simulink library "line_tracking_algorithm_atomic_sub_chart_library"  (R2013b)
settings: Solver=ode45  StartTime=0.0  StopTime=10.0  RelTol=1e-3
undefined symbols (not defined in the file): DiscIntNeverNeededParam, gcbh, realtime
libraries: legonxtlib x15, simulink x15
(part 2 of 2)

== system line_tracking_algorithm_atomic_sub_chart_library/line_tracking_mode1/line_tracking_mode.LineTrackAltFcn/D ==
  light error : Inport
  Abs1 : Abs
  Constant4 : Constant  Value=[2.5 0]  OutDataTypeStr=single
  Constant5 : Constant  Value=[0 1]  OutDataTypeStr=single
  Discrete Derivative1 : simulink/Discrete/Discrete Derivative  gainval=1.0  ICPrevScaledInput=0.0  InputProcessing=Inherited  OutMin=[]  OutMax=[]  OutDataTypeStr=single  OutputDataTypeScalingMode=single  OutDataType=fixdt(1, 16)  OutScaling=2^-10  DoSatur=off
  Gain2 : Gain  Gain=0.0005
  Low Pass Filter1 : DiscreteFilter  Numerator=[.2]  Denominator=[1 -0.8]
  Product1 : Product  RndMeth=Zero
  Switch1 : Switch
  Volt : Outport
  wires:
  light error/1 -> Low Pass Filter1/1
  Low Pass Filter1/1 -> Discrete Derivative1/1
  Abs1/1 -> Gain2/1
  Constant5/1 -> Switch1/3
  Constant4/1 -> Switch1/1
  Discrete Derivative1/1 -> Switch1/2, Abs1/1
  Switch1/1 -> Product1/1
  Gain2/1 -> Product1/2
  Product1/1 -> Volt/1

== system line_tracking_algorithm_atomic_sub_chart_library/line_tracking_mode1/line_tracking_mode.LineTrackAltFcn/LCD2 ==
  In1 : Inport
  Data Type Conversion : DataTypeConversion  OutDataTypeStr=int32
  LCD : S-Function  FunctionName=nxt_lcd  Parameters=lcdStr1, lcdLine, lcdFormat  EnableBusSupport=off  mask(NXT LCD){lcdStr=Lerror, lcdLine=5, lcdFormat=Decimal}
      mask prompts: lcdStr "Prefix String (MAX 8 Characters):"; lcdLine "Display at Line:"; lcdFormat "Display Format:"
      mask help: Displays a number on NXT LCD screen
      mask init:
      | lcdStr1= [uint8(lcdStr) uint8(0)];
      mask TypeOptions lcdLine: 1 | 2 | 3 | 4 | 5 | 6 | 7 | 8
      mask TypeOptions lcdFormat: Decimal | Hex
      mask Display:
      | color('blue');
      | text(0.65, 0.87, 'LEGO', 'horizontalAlignment', 'left');
      | color('black');
      | port_label('input', 1, '');
  wires:
  In1/1 -> Data Type Conversion/1
  Data Type Conversion/1 -> LCD/1

== system line_tracking_algorithm_atomic_sub_chart_library/line_tracking_mode1/line_tracking_mode.LineTrackAltFcn/P ==
  light Error : Inport
  Abs : Abs
  Constant2 : Constant  Value=[3 0]  OutDataTypeStr=single
  Constant3 : Constant  Value=[0 1]  OutDataTypeStr=single
  Gain4 : Gain  Gain=0.02
  Product : Product  RndMeth=Zero
  Switch : Switch
  Volt : Outport
  wires:
  light Error/1 -> Abs/1, Switch/2
  Switch/1 -> Product/1
  Constant3/1 -> Switch/3
  Constant2/1 -> Switch/1
  Abs/1 -> Gain4/1
  Gain4/1 -> Product/2
  Product/1 -> Volt/1

== system line_tracking_algorithm_atomic_sub_chart_library/line_tracking_mode1/line_tracking_mode.LineTrackAltFcn/Reference ==
  calib : Inport
  Bus Selector2 : BusSelector  OutputSignals=blackOnTail,whiteOnTail
  Gain : Gain  Gain=0.3
  Sum : Sum  Inputs=|+-
  Sum3 : Sum  Inputs=|++
  desired light : Outport
  wires:
  calib/1 -> Bus Selector2/1
  Bus Selector2/2 -> Sum3/2, Sum/2  "<whiteOnTail>"
  Bus Selector2/1 -> Sum/1  "<blackOnTail>"
  Sum/1 -> Gain/1
  Gain/1 -> Sum3/1
  Sum3/1 -> desired light/1

== system line_tracking_algorithm_atomic_sub_chart_library/line_tracking_mode_arch/line_tracking_mode.LineTrackAltFcn/Correction ==
  VLVR : Inport
  Abs1 : Abs
  Compare To Constant1 : simulink/Logic and Bit Operations/Compare To Constant  relop=>  const=100  OutDataTypeStr=boolean
  Correction For Saturation : Subsystem  TreatAsAtomicUnit=on
  Logical Operator : Logic  Operator=OR  Inputs=1  AllPortsSameDT=off  OutDataTypeStr=boolean
  Logical Operator1 : Logic  Operator=NOT  Inputs=1  AllPortsSameDT=off  OutDataTypeStr=boolean
  Merge : Merge
  Multiply : Product  Inputs=**
  No saturation : Subsystem  TreatAsAtomicUnit=on
  Sign : Signum
  VLVRSAT : Outport
  wires:
  VLVR/1 -> Sign/1, Abs1/1
  Abs1/1 -> No saturation/1(In1), Correction For Saturation/1(In1), Compare To Constant1/1
  Compare To Constant1/1 -> Logical Operator/1
  Logical Operator/1 -> Logical Operator1/1, Correction For Saturation/Enable
  Logical Operator1/1 -> No saturation/Enable
  Correction For Saturation/1(Out1) -> Merge/1
  No saturation/1(Out1) -> Merge/2
  Merge/1 -> Multiply/2
  Sign/1 -> Multiply/1
  Multiply/1 -> VLVRSAT/1

== system line_tracking_algorithm_atomic_sub_chart_library/line_tracking_mode_arch/line_tracking_mode.LineTrackAltFcn/D ==
  light error : Inport
  Abs1 : Abs
  Constant4 : Constant  Value=[3 0]  OutDataTypeStr=single
  Constant5 : Constant  Value=[0 1]  OutDataTypeStr=single
  Discrete Derivative1 : simulink/Discrete/Discrete Derivative  gainval=1.0  ICPrevScaledInput=0.0  InputProcessing=Inherited  OutMin=[]  OutMax=[]  OutDataTypeStr=single  OutputDataTypeScalingMode=single  OutDataType=fixdt(1, 16)  OutScaling=2^-10  DoSatur=off
  Gain2 : Gain  Gain=0.002
  Low Pass Filter1 : DiscreteFilter  Numerator=[.2]  Denominator=[1 -0.8]
  Product1 : Product  RndMeth=Zero
  Switch1 : Switch
  Volt : Outport
  wires:
  light error/1 -> Low Pass Filter1/1
  Low Pass Filter1/1 -> Discrete Derivative1/1
  Abs1/1 -> Gain2/1
  Constant5/1 -> Switch1/3
  Constant4/1 -> Switch1/1
  Discrete Derivative1/1 -> Switch1/2, Abs1/1
  Switch1/1 -> Product1/1
  Gain2/1 -> Product1/2
  Product1/1 -> Volt/1

== system line_tracking_algorithm_atomic_sub_chart_library/line_tracking_mode_arch/line_tracking_mode.LineTrackAltFcn/LCD2 ==
  In1 : Inport
  Data Type Conversion : DataTypeConversion  OutDataTypeStr=int32
  LCD : S-Function  FunctionName=nxt_lcd  Parameters=lcdStr1, lcdLine, lcdFormat  EnableBusSupport=off  mask(NXT LCD){lcdStr=Battery, lcdLine=8, lcdFormat=Decimal}
      mask prompts: lcdStr "Prefix String (MAX 8 Characters):"; lcdLine "Display at Line:"; lcdFormat "Display Format:"
      mask help: Displays a number on NXT LCD screen
      mask init:
      | lcdStr1= [uint8(lcdStr) uint8(0)];
      mask TypeOptions lcdLine: 1 | 2 | 3 | 4 | 5 | 6 | 7 | 8
      mask TypeOptions lcdFormat: Decimal | Hex
      mask Display:
      | color('blue');
      | text(0.65, 0.87, 'LEGO', 'horizontalAlignment', 'left');
      | color('black');
      | port_label('input', 1, '');
  wires:
  In1/1 -> Data Type Conversion/1
  Data Type Conversion/1 -> LCD/1

== system line_tracking_algorithm_atomic_sub_chart_library/line_tracking_mode_arch/line_tracking_mode.LineTrackAltFcn/P ==
  light Error : Inport
  Abs : Abs
  Constant2 : Constant  Value=[3 0]  OutDataTypeStr=single
  Constant3 : Constant  Value=[0 1]  OutDataTypeStr=single
  Gain4 : Gain  Gain=0.05
  Product : Product  RndMeth=Zero
  Switch : Switch
  Volt : Outport
  wires:
  light Error/1 -> Abs/1, Switch/2
  Switch/1 -> Product/1
  Constant3/1 -> Switch/3
  Constant2/1 -> Switch/1
  Abs/1 -> Gain4/1
  Gain4/1 -> Product/2
  Product/1 -> Volt/1

== system line_tracking_algorithm_atomic_sub_chart_library/line_tracking_mode_arch/line_tracking_mode.LineTrackAltFcn/Reference ==
  calib : Inport
  Bus Selector2 : BusSelector  OutputSignals=blackOnTail,whiteOnTail
  Gain : Gain  Gain=0.3
  Sum : Sum  Inputs=|+-
  Sum3 : Sum  Inputs=|++
  desired light : Outport
  wires:
  calib/1 -> Bus Selector2/1
  Bus Selector2/2 -> Sum3/2, Sum/2  "<whiteOnTail>"
  Bus Selector2/1 -> Sum/1  "<blackOnTail>"
  Sum/1 -> Gain/1
  Gain/1 -> Sum3/1
  Sum3/1 -> desired light/1

== system line_tracking_algorithm_atomic_sub_chart_library/line_tracking_mode_dev/line_tracking_mode.LineTrackAltFcn/Correction ==
  VLVR : Inport
  Abs1 : Abs
  Compare To Constant1 : simulink/Logic and Bit Operations/Compare To Constant  relop=>  const=100  OutDataTypeStr=boolean
  Correction For Saturation : Subsystem  TreatAsAtomicUnit=on
  Logical Operator : Logic  Operator=OR  Inputs=1  AllPortsSameDT=off  OutDataTypeStr=boolean
  Logical Operator1 : Logic  Operator=NOT  Inputs=1  AllPortsSameDT=off  OutDataTypeStr=boolean
  Merge : Merge
  Multiply : Product  Inputs=**
  No saturation : Subsystem  TreatAsAtomicUnit=on
  Sign : Signum
  VLVRSAT : Outport
  wires:
  VLVR/1 -> Sign/1, Abs1/1
  Abs1/1 -> No saturation/1(In1), Correction For Saturation/1(In1), Compare To Constant1/1
  Compare To Constant1/1 -> Logical Operator/1
  Logical Operator/1 -> Logical Operator1/1, Correction For Saturation/Enable
  Logical Operator1/1 -> No saturation/Enable
  Correction For Saturation/1(Out1) -> Merge/1
  No saturation/1(Out1) -> Merge/2
  Merge/1 -> Multiply/2
  Sign/1 -> Multiply/1
  Multiply/1 -> VLVRSAT/1

== system line_tracking_algorithm_atomic_sub_chart_library/line_tracking_mode_dev/line_tracking_mode.LineTrackAltFcn/D ==
  light error : Inport
  Abs1 : Abs
  Constant4 : Constant  Value=[3 0]  OutDataTypeStr=single
  Constant5 : Constant  Value=[0 1]  OutDataTypeStr=single
  Discrete Derivative1 : simulink/Discrete/Discrete Derivative  gainval=1.0  ICPrevScaledInput=0.0  InputProcessing=Inherited  OutMin=[]  OutMax=[]  OutDataTypeStr=single  OutputDataTypeScalingMode=single  OutDataType=fixdt(1, 16)  OutScaling=2^-10  DoSatur=off
  Gain2 : Gain  Gain=0.002
  Low Pass Filter1 : DiscreteFilter  Numerator=[.2]  Denominator=[1 -0.8]
  Product1 : Product  RndMeth=Zero
  Switch1 : Switch
  Volt : Outport
  wires:
  light error/1 -> Low Pass Filter1/1
  Low Pass Filter1/1 -> Discrete Derivative1/1
  Abs1/1 -> Gain2/1
  Constant5/1 -> Switch1/3
  Constant4/1 -> Switch1/1
  Discrete Derivative1/1 -> Switch1/2, Abs1/1
  Switch1/1 -> Product1/1
  Gain2/1 -> Product1/2
  Product1/1 -> Volt/1

== system line_tracking_algorithm_atomic_sub_chart_library/line_tracking_mode_dev/line_tracking_mode.LineTrackAltFcn/LCD2 ==
  In1 : Inport
  Data Type Conversion : DataTypeConversion  OutDataTypeStr=int32
  LCD : S-Function  FunctionName=nxt_lcd  Parameters=lcdStr1, lcdLine, lcdFormat  EnableBusSupport=off  mask(NXT LCD){lcdStr=Battery, lcdLine=8, lcdFormat=Decimal}
      mask prompts: lcdStr "Prefix String (MAX 8 Characters):"; lcdLine "Display at Line:"; lcdFormat "Display Format:"
      mask help: Displays a number on NXT LCD screen
      mask init:
      | lcdStr1= [uint8(lcdStr) uint8(0)];
      mask TypeOptions lcdLine: 1 | 2 | 3 | 4 | 5 | 6 | 7 | 8
      mask TypeOptions lcdFormat: Decimal | Hex
      mask Display:
      | color('blue');
      | text(0.65, 0.87, 'LEGO', 'horizontalAlignment', 'left');
      | color('black');
      | port_label('input', 1, '');
  wires:
  In1/1 -> Data Type Conversion/1
  Data Type Conversion/1 -> LCD/1

== system line_tracking_algorithm_atomic_sub_chart_library/line_tracking_mode_dev/line_tracking_mode.LineTrackAltFcn/P ==
  light Error : Inport
  Abs : Abs
  Constant2 : Constant  Value=[3 0]  OutDataTypeStr=single
  Constant3 : Constant  Value=[0 1]  OutDataTypeStr=single
  Gain4 : Gain  Gain=0.05
  Product : Product  RndMeth=Zero
  Switch : Switch
  Volt : Outport
  wires:
  light Error/1 -> Abs/1, Switch/2
  Switch/1 -> Product/1
  Constant3/1 -> Switch/3
  Constant2/1 -> Switch/1
  Abs/1 -> Gain4/1
  Gain4/1 -> Product/2
  Product/1 -> Volt/1

== system line_tracking_algorithm_atomic_sub_chart_library/line_tracking_mode_dev/line_tracking_mode.LineTrackAltFcn/Reference ==
  calib : Inport
  Bus Selector2 : BusSelector  OutputSignals=blackOnTail,whiteOnTail
  Gain : Gain  Gain=0.3
  Sum : Sum  Inputs=|+-
  Sum3 : Sum  Inputs=|++
  desired light : Outport
  wires:
  calib/1 -> Bus Selector2/1
  Bus Selector2/2 -> Sum3/2, Sum/2  "<whiteOnTail>"
  Bus Selector2/1 -> Sum/1  "<blackOnTail>"
  Sum/1 -> Gain/1
  Gain/1 -> Sum3/1
  Sum3/1 -> desired light/1

== system line_tracking_algorithm_atomic_sub_chart_library/line_tracking_mode_sid/line_tracking_mode.lineTrack/Direction ==
  In : Inport  OutDataTypeStr=boolean  PortDimensions=1
  Constant : Constant  Value=-1  OutDataTypeStr=single
  Constant1 : Constant  OutDataTypeStr=single
  Switch : Switch  Criteria=u2 ~= 0
  Out1 : Outport
  wires:
  Switch/1 -> Out1/1
  In/1 -> Switch/2
  Constant1/1 -> Switch/1
  Constant/1 -> Switch/3

== system line_tracking_algorithm_atomic_sub_chart_library/line_tracking_mode_sid/line_tracking_mode.lineTrack/LPF and deriv1 ==
  light : Inport
  Discrete Filter : DiscreteFilter  Numerator=[0.05]  Denominator=[1 -0.95]
  Gain : Gain  Gain=1/0.004
  Sum3 : Sum  Inputs=+-
  Unit Delay : UnitDelay  SampleTime=-1
  light_dot : Outport
  wires:
  Unit Delay/1 -> Sum3/2
  Gain/1 -> Unit Delay/1, Sum3/1
  Sum3/1 -> light_dot/1  "theta_dot_dot"
  Discrete Filter/1 -> Gain/1
  light/1 -> Discrete Filter/1

== system line_tracking_algorithm_atomic_sub_chart_library/line_tracking_mode_sid/line_tracking_mode.lineTrack/Saturation overshoot correction ==
  In1 : Inport
  Abs : Abs
  Bias : Bias  Bias=-100
  Compare To Constant : simulink/Logic and Bit Operations/Compare To Constant  relop=>  const=100  OutDataTypeStr=boolean
  Data Type Conversion : DataTypeConversion  OutDataTypeStr=single
  Multiply : Product  Inputs=***
  Sign : Signum
  Out1 : Outport
  wires:
  Sign/1 -> Multiply/1
  Abs/1 -> Compare To Constant/1, Bias/1
  In1/1 -> Abs/1, Sign/1
  Multiply/1 -> Out1/1
  Data Type Conversion/1 -> Multiply/3
  Bias/1 -> Multiply/2
  Compare To Constant/1 -> Data Type Conversion/1

== system line_tracking_algorithm_atomic_sub_chart_library/line_tracking_mode_sid/line_tracking_mode.lineTrack/deriv2 ==
  light_dot : Inport
  Sum3 : Sum  Inputs=+-
  Unit Delay : UnitDelay  SampleTime=-1
  lgiht_dot_dot : Outport
  wires:
  Sum3/1 -> lgiht_dot_dot/1  "lgiht_dot_dot"
  light_dot/1 -> Sum3/1, Unit Delay/1
  Unit Delay/1 -> Sum3/2

== system line_tracking_algorithm_atomic_sub_chart_library/line_tracking_limbo/line_tracking_mode.LineTrackAltFcn/Correction/Correction For Saturation ==
  In1 : Inport
  Enable : EnablePort
  Demux : Demux  Outputs=2
  Divide : Product  Inputs=/*
  Gain : Gain  Gain=100
  Gain1 : Gain  Gain=-1
  Saturation : Saturate  UpperLimit=100  LowerLimit=-100
  Sum : Sum  Inputs=-+|
  Switch : Switch
  Switch1 : Switch  Criteria=u2 > Threshold
  Switch2 : Switch
  Vector Concatenate : Concatenate
  Vector Concatenate1 : Concatenate
  Out1 : Outport
  wires:
  Switch2/1 -> Out1/1
  Vector Concatenate1/1 -> Switch2/3
  Vector Concatenate/1 -> Switch2/1
  Gain/1 -> Vector Concatenate1/1, Vector Concatenate/2
  Gain1/1 -> Switch1/2
  Divide/1 -> Gain/1
  Switch1/1 -> Divide/2
  Saturation/1 -> Vector Concatenate/1, Vector Concatenate1/2
  Switch/1 -> Saturation/1, Divide/1
  Sum/1 -> Switch/2, Switch2/2, Gain1/1
  Demux/2 -> Switch/3, Switch1/3, Sum/1
  Demux/1 -> Switch/1, Switch1/1, Sum/2
  In1/1 -> Demux/1

== system line_tracking_algorithm_atomic_sub_chart_library/line_tracking_limbo/line_tracking_mode.LineTrackAltFcn/Correction/No saturation ==
  In1 : Inport
  Enable : EnablePort
  Out1 : Outport
  wires:
  In1/1 -> Out1/1

== system line_tracking_algorithm_atomic_sub_chart_library/line_tracking_mode/line_tracking_mode.LineTrackAltFcn/Correction/Correction For Saturation ==
  In1 : Inport
  Enable : EnablePort
  Demux : Demux  Outputs=2
  Divide : Product  Inputs=/*
  Gain : Gain  Gain=100
  Gain1 : Gain  Gain=-1
  Saturation : Saturate  UpperLimit=100  LowerLimit=-100
  Sum : Sum  Inputs=-+|
  Switch : Switch
  Switch1 : Switch  Criteria=u2 > Threshold
  Switch2 : Switch
  Vector Concatenate : Concatenate
  Vector Concatenate1 : Concatenate
  Out1 : Outport
  wires:
  Switch2/1 -> Out1/1
  Vector Concatenate1/1 -> Switch2/3
  Vector Concatenate/1 -> Switch2/1
  Gain/1 -> Vector Concatenate1/1, Vector Concatenate/2
  Gain1/1 -> Switch1/2
  Divide/1 -> Gain/1
  Switch1/1 -> Divide/2
  Saturation/1 -> Vector Concatenate/1, Vector Concatenate1/2
  Switch/1 -> Saturation/1, Divide/1
  Sum/1 -> Switch/2, Switch2/2, Gain1/1
  Demux/2 -> Switch/3, Switch1/3, Sum/1
  Demux/1 -> Switch/1, Switch1/1, Sum/2
  In1/1 -> Demux/1

== system line_tracking_algorithm_atomic_sub_chart_library/line_tracking_mode/line_tracking_mode.LineTrackAltFcn/Correction/No saturation ==
  In1 : Inport
  Enable : EnablePort
  Out1 : Outport
  wires:
  In1/1 -> Out1/1

== system line_tracking_algorithm_atomic_sub_chart_library/line_tracking_mode_arch/line_tracking_mode.LineTrackAltFcn/Correction/Correction For Saturation ==
  In1 : Inport
  Enable : EnablePort
  Demux : Demux  Outputs=2
  Divide : Product  Inputs=/*
  Gain : Gain  Gain=100
  Gain1 : Gain  Gain=-1
  Saturation : Saturate  UpperLimit=100  LowerLimit=-100
  Sum : Sum  Inputs=-+|
  Switch : Switch
  Switch1 : Switch  Criteria=u2 > Threshold
  Switch2 : Switch
  Vector Concatenate : Concatenate
  Vector Concatenate1 : Concatenate
  Out1 : Outport
  wires:
  In1/1 -> Demux/1
  Demux/1 -> Sum/2, Switch1/1, Switch/1
  Demux/2 -> Sum/1, Switch1/3, Switch/3
  Sum/1 -> Gain1/1, Switch2/2, Switch/2
  Switch/1 -> Divide/1, Saturation/1
  Saturation/1 -> Vector Concatenate1/2, Vector Concatenate/1
  Switch1/1 -> Divide/2
  Divide/1 -> Gain/1
  Gain1/1 -> Switch1/2
  Gain/1 -> Vector Concatenate/2, Vector Concatenate1/1
  Vector Concatenate/1 -> Switch2/1
  Vector Concatenate1/1 -> Switch2/3
  Switch2/1 -> Out1/1

== system line_tracking_algorithm_atomic_sub_chart_library/line_tracking_mode_arch/line_tracking_mode.LineTrackAltFcn/Correction/No saturation ==
  In1 : Inport
  Enable : EnablePort
  Out1 : Outport
  wires:
  In1/1 -> Out1/1

== system line_tracking_algorithm_atomic_sub_chart_library/line_tracking_mode_dev/line_tracking_mode.LineTrackAltFcn/Correction/Correction For Saturation ==
  In1 : Inport
  Enable : EnablePort
  Demux : Demux  Outputs=2
  Divide : Product  Inputs=/*
  Gain : Gain  Gain=100
  Gain1 : Gain  Gain=-1
  Saturation : Saturate  UpperLimit=100  LowerLimit=-100
  Sum : Sum  Inputs=-+|
  Switch : Switch
  Switch1 : Switch  Criteria=u2 > Threshold
  Switch2 : Switch
  Vector Concatenate : Concatenate
  Vector Concatenate1 : Concatenate
  Out1 : Outport
  wires:
  In1/1 -> Demux/1
  Demux/1 -> Sum/2, Switch1/1, Switch/1
  Demux/2 -> Sum/1, Switch1/3, Switch/3
  Sum/1 -> Gain1/1, Switch2/2, Switch/2
  Switch/1 -> Divide/1, Saturation/1
  Saturation/1 -> Vector Concatenate1/2, Vector Concatenate/1
  Switch1/1 -> Divide/2
  Divide/1 -> Gain/1
  Gain1/1 -> Switch1/2
  Gain/1 -> Vector Concatenate/2, Vector Concatenate1/1
  Vector Concatenate/1 -> Switch2/1
  Vector Concatenate1/1 -> Switch2/3
  Switch2/1 -> Out1/1

== system line_tracking_algorithm_atomic_sub_chart_library/line_tracking_mode_dev/line_tracking_mode.LineTrackAltFcn/Correction/No saturation ==
  In1 : Inport
  Enable : EnablePort
  Out1 : Outport
  wires:
  In1/1 -> Out1/1

== stateflow chart line_tracking_algorithm_atomic_sub_chart_library/line_tracking_mode ==
  state line_tracking_mode
    entry:
    desired_tail = single(1.6); %radian
    entry, during:
    PWM.tail = tail_controller(sensors.theta_T,desired_tail);
    state Waiting
      entry: debugFlag = uint16(400);
    state Track
      entry:
      debugFlag = uint16(401);
      speed_ref = single(45);
      during:
      [desired_tail, PWM.left, PWM.right] = LineTrackAltFcn(sensors,lightCalib,states,speed_ref)
      state Race
        during:
        DispTheta(states.balancerStates.theta);
      state Decelerate
        during:
        speed_ref = speed_ref - single(0.1);
      (default) -> Race
      Race -> Decelerate : [states.balancerStates.theta > single(441)]
    state Done
      entry:
      debugFlag = uint16(402);
      PWM.left = single(0); PWM.right = single(0);
      current_mode_status = OperationModeStatusEnum.SUCCESSFULLY_COMPLETED;
    state DispTheta(theta) [function]
    state [V_left,V_right] = lineTrack(light,lightCalib,forwardSpeed) [function]
    state cmd = tail_controller(current,desired) [function]
    state [tail,PWM_left,PWM_right] = LineTrackAltFcn(sensors,lightCalib,states,forwardSpeed) [function]
    (default) -> Waiting
    Waiting -> Track : [hasChangedFrom(touch,single(0))]
    Decelerate -> Done : [speed_ref<single(0)]
  data: theta function_input double size=1; light function_input single size=1; lightCalib function_input Bus: Light_Bus size=1; V_left function_output single size=1; V_right function_output single size=1; forwardSpeed function_input single size=1; current function_input single size=1; desired function_input single size=1; cmd function_output single size=1; tail function_output single; sensors function_input Bus: Sensors_Bus size=1; lightCalib function_input Bus: Light_Bus size=1; states function_input Bus: States_Bus size=1; PWM_left function_output single; PWM_right function_output single; forwardSpeed function_input single size=1; sensors input Bus: Sensors_Bus size=1; lightCalib data_store_memory size=1; touch input single size=1; PWM output Bus: PWM_bus size=1; debugFlag output uint16 size=1; current_mode_status data_store_memory; desired_tail local single size=1; speed_ref local single size=1; states input Bus: States_Bus size=1

== stateflow chart line_tracking_algorithm_atomic_sub_chart_library/line_tracking_mode1 ==
  state line_tracking_mode
    entry:
    desired_tail = single(1.6); %radian
    during:
    PWM.tail = tail_controller(sensors.theta_T,desired_tail);
    state Waiting
      entry: debugFlag = uint16(400);
    state Track
      entry:
      debugFlag = uint16(401);
      speed_ref = single(40);
      during:
      [desired_tail, PWM.left, PWM.right] = LineTrackAltFcn(sensors,lightCalib,states.balancerStates,speed_ref)
      state Race
        during:
        DispTheta(states.balancerStates.theta);
      state Decelerate
        during:
        speed_ref = speed_ref - single(0.1);
      (default) -> Race
      Race -> Decelerate : [states.balancerStates.theta > single(450)]
    state Done
      entry:
      debugFlag = uint16(402);
      PWM.left = single(0); PWM.right = single(0);
      current_mode_status = OperationModeStatusEnum.SUCCESSFULLY_COMPLETED;
    state DispTheta(theta) [function]
    state [V_left,V_right] = lineTrack(light,lightCalib,forwardSpeed) [function]
    state cmd = tail_controller(current,desired) [function]
    state [tail,PWM_left,PWM_right] = LineTrackAltFcn(sensors,lightCalib,states,forwardSpeed) [function]
    (default) -> Waiting
    Waiting -> Track : [hasChangedFrom(touch,single(0))]
    Decelerate -> Done : [speed_ref<single(0)]
  data: theta function_input double size=1; light function_input single size=1; lightCalib function_input Bus: Light_Bus size=1; V_left function_output single size=1; V_right function_output single size=1; forwardSpeed function_input single size=1; current function_input single size=1; desired function_input single size=1; cmd function_output single size=1; tail function_output single; sensors function_input Bus: Sensors_Bus size=1; lightCalib function_input Bus: Light_Bus size=1; states function_input Bus: Balancer_States_Bus size=1; PWM_left function_output single; PWM_right function_output single; forwardSpeed function_input single size=1; sensors input Bus: Sensors_Bus size=1; lightCalib data_store_memory size=1; touch input single size=1; PWM output Bus: PWM_bus size=1; debugFlag output uint16 size=1; current_mode_status data_store_memory; desired_tail local single size=1; speed_ref local single size=1; states input Bus: States_Bus size=1

== stateflow chart line_tracking_algorithm_atomic_sub_chart_library/line_tracking_mode_arch ==
  state line_tracking_mode
    entry:
    desired_tail = single(1.6); %radian
    entry, during:
    PWM.tail = tail_controller(sensors.theta_T,desired_tail);
    state Waiting
      entry: debugFlag = uint16(400);
    state Track
      entry:
      debugFlag = uint16(401);
      speed_ref = single(45);
      during:
      [desired_tail, PWM.left, PWM.right] = LineTrackAltFcn(sensors,lightCalib,states,speed_ref)
      state Race
        during:
        %DispTheta(states.balancerStates.theta);
      state Decelerate
        during:
        speed_ref = speed_ref - single(0.1);
      (default) -> Race
      Race -> Decelerate : [states.balancerStates.theta > single(325)]
    state Done
      entry:
      debugFlag = uint16(402);
      PWM.left = single(0); PWM.right = single(0);
      current_mode_status = OperationModeStatusEnum.SUCCESSFULLY_COMPLETED;
    state [V_left,V_right] = lineTrack(light,lightCalib,forwardSpeed) [function]
    state cmd = tail_controller(current,desired) [function]
    state [tail,PWM_left,PWM_right] = LineTrackAltFcn(sensors,lightCalib,states,forwardSpeed) [function]
    (default) -> Waiting
    Waiting -> Track : [hasChangedFrom(touch,single(0))]
    Decelerate -> Done : [speed_ref<single(0)]
  data: light function_input single size=1; lightCalib function_input Bus: Light_Bus size=1; V_left function_output single size=1; V_right function_output single size=1; forwardSpeed function_input single size=1; current function_input single size=1; desired function_input single size=1; cmd function_output single size=1; tail function_output single; sensors function_input Bus: Sensors_Bus size=1; lightCalib function_input Bus: Light_Bus size=1; states function_input Bus: States_Bus size=1; PWM_left function_output single; PWM_right function_output single; forwardSpeed function_input single size=1; sensors input Bus: Sensors_Bus size=1; lightCalib data_store_memory size=1; touch input single size=1; PWM output Bus: PWM_bus size=1; debugFlag output uint16 size=1; current_mode_status data_store_memory; desired_tail local single size=1; speed_ref local single size=1; states input Bus: States_Bus size=1

== stateflow chart line_tracking_algorithm_atomic_sub_chart_library/line_tracking_mode_sid ==
  state line_tracking_mode
    entry:
    desired_tail = single(1.6); %radian
    during:
    PWM.tail = tail_controller(sensors.theta_T,desired_tail);
    state Waiting
      entry: debugFlag = uint16(400);
    state Track
      entry:
      DirectionRight=false;
      Event_Search=false;
      Speed=single(65);
      during:
      CalibratedLight=CalibrateLight(sensors.light,lightCalib);
      state RecalculateLOrR
        entry:
        orig_phi=states.phi;
        turningPWM=single(0);
        fov=single(0);
        during:
        PWM.left = fov+turningPWM;
        PWM.right = fov-turningPWM;
        state TurnLeft
          entry:
          debugFlag = uint16(422);
          desired_phi=orig_phi;
          during:
          desired_phi=desired_phi+single(0.008);
          turningPWM= phiController(states.phi,desired_phi,sensors.battery);
        state TurnRight
          entry:
          debugFlag = uint16(423);
          during:
          desired_phi=desired_phi-single(0.008);
          turningPWM= phiController(states.phi,desired_phi,sensors.battery);
        state GoBack
          entry:
          debugFlag = uint16(463);
          count=uint16(0);
          during:
          turningPWM= single(0);
          fov=single(-50);
          count=count+uint16(1);
        state GoBackToOriginalPosition
          entry:
          debugFlag = uint16(424);
          during:
          desired_phi=desired_phi+single(0.008);
          turningPWM= phiController(states.phi,desired_phi,sensors.battery);
        state FindLineNow
          entry:
          debugFlag = uint16(425);
          during:
          [PWM.left, PWM.right, ~] = lineTrack(CalibratedLight, DirectionRight, 2/3*Speed)
        (default) -> TurnLeft
        GoBack -> TurnLeft : [count>500]
        TurnLeft -> (junction 77) : [(states.phi-orig_phi)>single(0.5)]
        (junction 77) -> TurnRight : {TempLight=CalibratedLight;}
        TurnRight -> (junction 79) : [(states.phi-orig_phi)<single(-0.5)]
        (junction 79) -> GoBack [order 1] : [abs(TempLight-CalibratedLight)>0.08]
        (junction 79) -> (junction 94) [order 2] : {DirectionRight=TempLight>CalibratedLight}
        (junction 94) -> GoBackToOriginalPosition [order 1] : [DirectionRight==1]
        (junction 94) -> FindLineNow [order 2] : [DirectionRight==0]
        GoBackToOriginalPosition -> FindLineNow : [(states.phi-orig_phi)>0]
      state CaptureLine
        entry:
        Event_Search=false;
        count=uint16(0);
        countCapture=uint16(0);
        SearchCount=single(0);
        during:
        countCapture=countCapture+uint16(1);
        if (SearchCount>single(40))
        Event_Search=true;
        else
        if(CalibratedLight<0.01)
        SearchCount=SearchCount+single(1);
        else
        Event_Search=false;
        SearchCount=single(0);
        end
        end
        state TrackNormally2
          entry:
          debugFlag = uint16(441);
          swap=false;
          during:
          [PWM.left, PWM.right, swap] = lineTrack(CalibratedLight, DirectionRight, single(40));
        state ConfirmDirectionSwap2
          entry:
          debugFlag = uint16(442);
          count=uint16(0);
          during:
          [PWM.left, PWM.right, swap] = lineTrack(CalibratedLight, DirectionRight, single(40));
          count=count+uint16(1);
        (default) -> TrackNormally2
        ConfirmDirectionSwap2 -> TrackNormally2 [order 1] : [count>=uint16(5+15*(50/(1+Speed)))]
            | {DirectionRight=~DirectionRight; Speak}
        ConfirmDirectionSwap2 -> TrackNormally2 [order 2] : [swap==false]
        TrackNormally2 -> ConfirmDirectionSwap2 : [swap==true&&CalibratedLight>0.01]
      state FollowEdge
        entry:
        Event_Search=false;
        count=uint16(0);
        SearchCount=single(0);
        during:
        if (SearchCount>single(40))
        Event_Search=true;
        else
        if(CalibratedLight<0.01)
        SearchCount=SearchCount+single(1);
        else
        Event_Search=false;
        SearchCount=single(0);
        end
        end
        state TrackNormally
          entry:
          debugFlag = uint16(411);
          swap=false;
          during:
          [PWM.left, PWM.right, swap] = lineTrack(CalibratedLight, DirectionRight, Speed);
        state ConfirmDirectionSwap
          entry:
          debugFlag = uint16(412);
          count=uint16(0);
          during:
          [PWM.left, PWM.right, swap] = lineTrack(CalibratedLight, DirectionRight, Speed);
          count=count+uint16(1);
        (default) -> TrackNormally
        ConfirmDirectionSwap -> TrackNormally [order 1] : [count>=uint16(5+15*(50/(1+Speed)))]
            | {DirectionRight=~DirectionRight; Speak}
        ConfirmDirectionSwap -> TrackNormally [order 2] : [swap==false]
        TrackNormally -> ConfirmDirectionSwap : [swap==true&&CalibratedLight>0.01]
      RecalculateLOrR -> CaptureLine : [CalibratedLight>0.2]
      CaptureLine -> RecalculateLOrR [order 1] : [Event_Search==true]
      FollowEdge -> RecalculateLOrR : [Event_Search==true]
      CaptureLine -> FollowEdge [order 2] : [countCapture>500]
      (default) -> FollowEdge
    state Done
      entry:
      debugFlag = uint16(404);
      PWM.left = single(0); PWM.right = single(0);
      current_mode_status = OperationModeStatusEnum.SUCCESSFULLY_COMPLETED;
    state [V_left,V_right,swap] = lineTrack(CalibrateLight,DirectionRight,Speed) [function]
    state CalibratedLight = CalibrateLight(light,lightCalib) [function]
    state Speak [function]
    state cmd = phiController(phi,desiredPhi,battery) [function]
    state cmd = tail_controller(current,desired) [function]
    (default) -> Waiting
    Waiting -> Track : [hasChangedFrom(touch,single(0))]
    Track -> Done : [hasChangedFrom(touch,single(0))]
  data: desired_phi local single size=1; orig_phi local single size=1; TempLight local single size=1; count local uint16 size=1; fov local single size=1; swap local boolean size=1; count local uint16 size=1; SearchCount local single size=1; swap local boolean size=1; count local uint16 size=1; SearchCount local single size=1; CalibratedLight local single size=1; Event_Search local boolean size=1; Speed local single size=1; countCapture local uint16 size=1; V_left function_output single size=1; V_right function_output single size=1; swap function_output boolean size=1; CalibrateLight function_input single size=1; DirectionRight function_input boolean size=1; Speed function_input single size=1; light function_input single size=1; lightCalib function_input Bus: Light_Bus size=1; CalibratedLight function_output single; cmd function_output single; phi function_input single size=1; desiredPhi function_input single size=1; battery function_input double size=1; current function_input single size=1; desired function_input single size=1; cmd function_output single size=1; sensors input Bus: Sensors_Bus size=1; lightCalib data_store_memory size=1; touch input single size=1; PWM output Bus: PWM_bus size=1; debugFlag output uint16 size=1; current_mode_status data_store_memory; desired_tail local single size=1; states input Bus: States_Bus size=1; DirectionRight local boolean size=1; turningPWM local single size=1

== stateflow chart line_tracking_algorithm_atomic_sub_chart_library/line_tracking_mode_dev ==
  state line_tracking_mode
    entry:
    desired_tail = single(1.6); %radian
    entry, during:
    PWM.tail = tail_controller(sensors.theta_T,desired_tail);
    state Waiting
      entry: debugFlag = uint16(400);
    state Track
      entry:
      debugFlag = uint16(401);
      speed_ref = single(45);
      during:
      [desired_tail, PWM.left, PWM.right] = LineTrackAltFcn(sensors,lightCalib,states,speed_ref)
      state Race
        during:
        DispTheta(states.balancerStates.theta);
      state Decelerate
        during:
        speed_ref = speed_ref - single(0.1);
      (default) -> Race
      Race -> Decelerate : [states.balancerStates.theta > single(441)]
    state Done
      entry:
      debugFlag = uint16(402);
      PWM.left = single(0); PWM.right = single(0);
      current_mode_status = OperationModeStatusEnum.SUCCESSFULLY_COMPLETED;
    state DispTheta(theta) [function]
    state [V_left,V_right] = lineTrack(light,lightCalib,forwardSpeed) [function]
    state cmd = tail_controller(current,desired) [function]
    state [tail,PWM_left,PWM_right] = LineTrackAltFcn(sensors,lightCalib,states,forwardSpeed) [function]
    (default) -> Waiting
    Waiting -> Track : [sensors.BT_status_in == single(11)]
    Decelerate -> Done : [speed_ref<single(0)]
  data: theta function_input double size=1; light function_input single size=1; lightCalib function_input Bus: Light_Bus size=1; V_left function_output single size=1; V_right function_output single size=1; forwardSpeed function_input single size=1; current function_input single size=1; desired function_input single size=1; cmd function_output single size=1; tail function_output single; sensors function_input Bus: Sensors_Bus size=1; lightCalib function_input Bus: Light_Bus size=1; states function_input Bus: States_Bus size=1; PWM_left function_output single; PWM_right function_output single; forwardSpeed function_input single size=1; sensors input Bus: Sensors_Bus size=1; lightCalib data_store_memory size=1; touch input single size=1; PWM output Bus: PWM_bus size=1; debugFlag output uint16 size=1; current_mode_status data_store_memory; desired_tail local single size=1; speed_ref local single size=1; states input Bus: States_Bus size=1

== stateflow chart line_tracking_algorithm_atomic_sub_chart_library/line_tracking_limbo ==
  state line_tracking_mode
    entry:
    desired_tail = single(1.6); %radian
    entry, during:
    PWM.tail = tail_controller(sensors.theta_T,desired_tail);
    state Waiting
      entry: debugFlag = uint16(400);
    state Track
      entry:
      debugFlag = uint16(401);
      speed_ref = single(45);
      during:
      [desired_tail, PWM.left, PWM.right] = LineTrackAltFcn(sensors,lightCalib,states,speed_ref)
      state Race
        during:
        DispTheta(states.balancerStates.theta);
      state Decelerate
        during:
        speed_ref = speed_ref - single(0.1);
      (default) -> Race
      Race -> Decelerate : [states.balancerStates.theta > single(425)]
    state Done
      entry:
      debugFlag = uint16(402);
      PWM.left = single(0); PWM.right = single(0);
      current_mode_status = OperationModeStatusEnum.SUCCESSFULLY_COMPLETED;
    state DispTheta(theta) [function]
    state [V_left,V_right] = lineTrack(light,lightCalib,forwardSpeed) [function]
    state cmd = tail_controller(current,desired) [function]
    state [tail,PWM_left,PWM_right] = LineTrackAltFcn(sensors,lightCalib,states,forwardSpeed) [function]
    (default) -> Waiting
    Waiting -> Track : [sensors.BT_status_in == single(11)]
    Decelerate -> Done : [speed_ref<single(0)]
  data: theta function_input double size=1; light function_input single size=1; lightCalib function_input Bus: Light_Bus size=1; V_left function_output single size=1; V_right function_output single size=1; forwardSpeed function_input single size=1; current function_input single size=1; desired function_input single size=1; cmd function_output single size=1; tail function_output single; sensors function_input Bus: Sensors_Bus size=1; lightCalib function_input Bus: Light_Bus size=1; states function_input Bus: States_Bus size=1; PWM_left function_output single; PWM_right function_output single; forwardSpeed function_input single size=1; sensors input Bus: Sensors_Bus size=1; lightCalib data_store_memory size=1; touch input single size=1; PWM output Bus: PWM_bus size=1; debugFlag output uint16 size=1; current_mode_status data_store_memory; desired_tail local single size=1; speed_ref local single size=1; states input Bus: States_Bus size=1
